simulink library "csu_slh_slosh"  (R2014b)
settings: Solver=ode45  StartTime=0.0  StopTime=10.0  RelTol=1e-3
libraries: util_slosh_lib x4
settings Model: Creator=Mark Agbayani  LastModifiedBy=Mark Agbayani

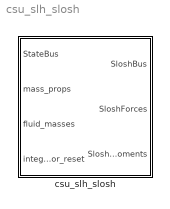
== system csu_slh_slosh ==
  csu_slh_slosh : Subsystem

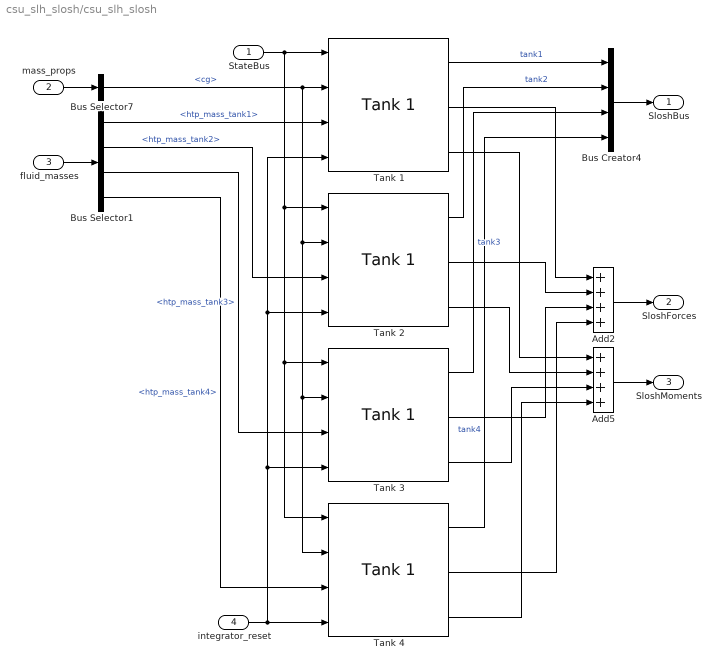
== system csu_slh_slosh/csu_slh_slosh ==
  StateBus : Inport
  mass_props : Inport  Port=2
  fluid_masses : Inport  Port=3
  integrator_reset : Inport  Port=4
  Add2 : Sum  Inputs=++++
  Add5 : Sum  Inputs=++++
  Bus Creator4 : BusCreator
  Bus Selector1 : BusSelector  OutputSignals=htp_mass_tank1,htp_mass_tank2,htp_mass_tank3,htp_mass_tank4
  Bus Selector7 : BusSelector  OutputSignals=cg
  Tank 1 : util_slosh_lib/Tank 1  forces_enable=slh_forces_enable  moments_enable=slh_moments_enable  damping_enable=slh_damping_enable  phi_2dot_limit=slh_htp_phi_2dot_limit  mass_fillfrac_100=mpl_htp_mass_fillfrac_100  tank_radius=mpl_htp_tank_radius  tank_center=mpl_htp_center_tank1  IC_settle_time=slh_IC_settle_time
  Tank 2 : util_slosh_lib/Tank 1  forces_enable=slh_forces_enable  moments_enable=slh_moments_enable  damping_enable=slh_damping_enable  phi_2dot_limit=slh_htp_phi_2dot_limit  mass_fillfrac_100=mpl_htp_mass_fillfrac_100  tank_radius=mpl_htp_tank_radius  tank_center=mpl_htp_center_tank2  IC_settle_time=slh_IC_settle_time
  Tank 3 : util_slosh_lib/Tank 1  forces_enable=slh_forces_enable  moments_enable=slh_moments_enable  damping_enable=slh_damping_enable  phi_2dot_limit=slh_htp_phi_2dot_limit  mass_fillfrac_100=mpl_htp_mass_fillfrac_100  tank_radius=mpl_htp_tank_radius  tank_center=mpl_htp_center_tank3  IC_settle_time=slh_IC_settle_time
  Tank 4 : util_slosh_lib/Tank 1  forces_enable=slh_forces_enable  moments_enable=slh_moments_enable  damping_enable=slh_damping_enable  phi_2dot_limit=slh_htp_phi_2dot_limit  mass_fillfrac_100=mpl_htp_mass_fillfrac_100  tank_radius=mpl_htp_tank_radius  tank_center=mpl_htp_center_tank4  IC_settle_time=slh_IC_settle_time
  SloshBus : Outport
  SloshForces : Outport  Port=2
  SloshMoments : Outport  Port=3
  wires:
  Tank 4/1 -> Bus Creator4/4  "tank4"
  Tank 3/1 -> Bus Creator4/3  "tank3"
  Tank 2/1 -> Bus Creator4/2  "tank2"
  Bus Creator4/1 -> SloshBus/1
  Tank 1/1 -> Bus Creator4/1  "tank1"
  fluid_masses/1 -> Bus Selector1/1
  mass_props/1 -> Bus Selector7/1
  StateBus/1 -> Tank 3/1, Tank 4/1, Tank 2/1, Tank 1/1
  Tank 4/3 -> Add5/4
  Tank 3/3 -> Add5/3
  Tank 2/3 -> Add5/2
  Tank 4/2 -> Add2/4
  Tank 3/2 -> Add2/3
  Tank 2/2 -> Add2/2
  Add5/1 -> SloshMoments/1
  Add2/1 -> SloshForces/1
  Bus Selector7/1 -> Tank 3/2, Tank 4/2, Tank 2/2, Tank 1/2  "<cg>"
  Bus Selector1/2 -> Tank 2/3  "<htp_mass_tank2>"
  Bus Selector1/3 -> Tank 3/3  "<htp_mass_tank3>"
  Bus Selector1/4 -> Tank 4/3  "<htp_mass_tank4>"
  Bus Selector1/1 -> Tank 1/3  "<htp_mass_tank1>"
  integrator_reset/1 -> Tank 1/4, Tank 2/4, Tank 3/4, Tank 4/4
  Tank 1/3 -> Add5/1
  Tank 1/2 -> Add2/1
